simulink model "problem4"  (R2020b)
settings: Solver=VariableStepAuto  StartTime=0.0  StopTime=10.0  RelTol=1e-3
model workspace (MAT data in the model file):
  J = Simulink.Parameter
  J.Value = 3
  J.DataType = 'auto'
  J.Dimensions = [1 1]
  K = Simulink.Parameter
  K.Value = 30
  K.DataType = 'auto'
  K.Dimensions = [1 1]
  Kd = Simulink.Parameter
  Kd.Value = 20
  Kd.DataType = 'auto'
  Kd.Dimensions = [1 1]
  Ki = Simulink.Parameter
  Ki.Value = 100
  Ki.DataType = 'auto'
  Ki.Dimensions = [1 1]
  Kp = Simulink.Parameter
  Kp.Value = 10
  Kp.DataType = 'auto'
  Kp.Dimensions = [1 1]
  L = Simulink.Parameter
  L.Value = 5
  L.DataType = 'auto'
  L.Dimensions = [1 1]
  R = Simulink.Parameter
  R.Value = 2
  R.DataType = 'auto'
  R.Dimensions = [1 1]
  b = Simulink.Parameter
  b.Value = 50
  b.DataType = 'auto'
  b.Dimensions = [1 1]
settings Model: Creator=admin  LastModifiedBy=admin

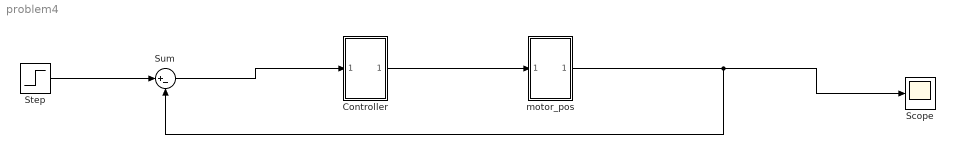
== system problem4 ==
  Controller : Subsystem
  Scope : Scope
  Step : Step  SampleTime=0
  Sum : Sum  Inputs=|+-
  motor_pos : ModelReference  ModelNameDialog=motor_pos  ModelReferenceVersion=1.1
  wires:
  motor_pos/1 -> Sum/2, Scope/1
  Controller/1(Out1) -> motor_pos/1
  Step/1 -> Sum/1
  Sum/1 -> Controller/1(In1)

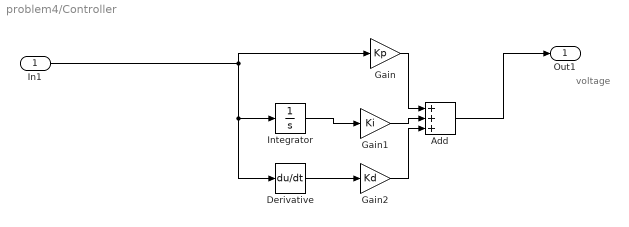
== system problem4/Controller ==
  note: voltage
  In1 : Inport
  Add : Sum  Inputs=+++
  Derivative : Derivative
  Gain : Gain  Gain=Kp
  Gain1 : Gain  Gain=Ki
  Gain2 : Gain  Gain=Kd
  Integrator : Integrator
  Out1 : Outport
  wires:
  In1/1 -> Derivative/1, Integrator/1, Gain/1
  Gain2/1 -> Add/3
  Gain1/1 -> Add/2
  Integrator/1 -> Gain1/1
  Add/1 -> Out1/1
  Derivative/1 -> Gain2/1
  Gain/1 -> Add/1
